simulink model "multififo"  (R2012b)
settings: Solver=ode45  StartTime=0.0  StopTime=40000  RelTol=1e-3
libraries: xbsIndex_r4 x136, xps_library x1
settings Model: Creator=tmadden  LastModifiedBy=tmadden

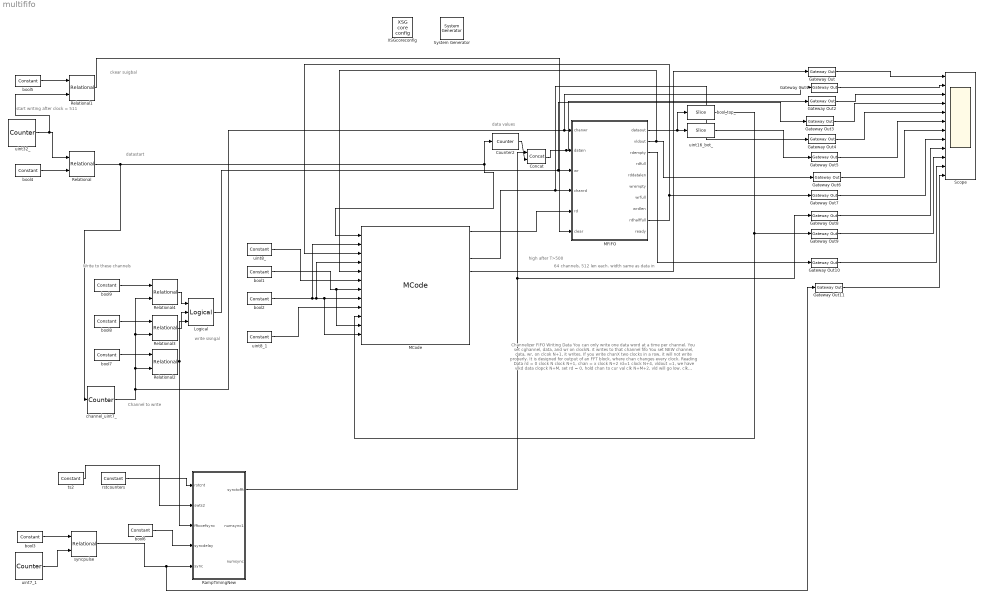
== system multififo ==
  note: Write to these channels
  note: write sisngal
  note: Channel to write
  note: data values
  note: ckear suigbal
  note: datastart
  note: start writing after clock = 511
  note: Channelizer FIFO
      | Writing Data
      | You can only write one data word at a time per channel.
      | You set cghannel, data, and wr on clockN. it writes to that channel fifo
      | You set NEW channel, data, wr, on clcok N+1, it writes.
      | If you write chanX two clocks in a row, it will not write properly.
      | It is designed for output of an FFT block, where chan changes every clock.
      |
      |
      | Reading Data
      | rd = 0 clock N
      | clock N+1, chan = x
      | clock N+2 rd=1
      | clock N+4, vldout =1, we have vlkd data
      | clopck N+M, set rd = 0, hold chan to cur val
      |
      | clk N+M+2, vld will go low.
      | clk N+M+3, chan  = new channel
      | clk N+M+4, rd=1
      | clk N+M+6, vld will be hi w/ new data
      |
      | You cannot read differnet channels per clock. you must read many data per clock,
      | at least 4 clks, so chan changes w./ rd off, and you waot for vld to go hi, 2 clkcs later.
  note: high after T>500
  note: 64 channels, 512 len each. width same as data in
  " System Generator" : xbsIndex_r4/ System Generator  Tag=genX  xilinxfamily=Kintex7  part=xc7k325t  speed=-3  package=fbg676  synthesis_tool=XST  clock_wrapper=Clock Enables  directory=./netlist  proj_type=Project Navigator  Synth_file=XST Defaults  Impl_file=ISE Defaults  testbench=off  simulink_period=1  sysclk_period=10  dcm_input_clock_period=10  incr_netlist=off  trim_vbits=Everywhere in SubSystem  dbl_ovrd=According to Block Masks  core_generation=According to Block Masks  run_coregen=off  deprecated_control=off  eval_field=0  block_type=sysgen
  Concat : xbsIndex_r4/Concat  num_inputs=2  dbl_ovrd=off  block_type=concat
  Counter2 : xbsIndex_r4/Counter  cnt_type=Free Running  cnt_to=4  operation=Up  start_count=0  cnt_by_val=1  arith_type=Unsigned  n_bits=16  bin_pt=0  load_pin=off  rst=off  en=on  explicit_period=on  period=1  dbl_ovrd=off  use_behavioral_HDL=off  implementation=Fabric  block_type=counter
  Gateway Out{,1..11} (12 alike) : xbsIndex_r4/Gateway Out  inherit_from_input=off  hdl_port=on  timing_constraint=None  locs_specified=off  LOCs={}  UseAsDAC=off  DACChannel='1'  block_type=gatewayout
  Logical : xbsIndex_r4/Logical  logical_function=OR  inputs=3  en=off  latency=0  precision=Full  arith_type=Unsigned  n_bits=16  bin_pt=0  align_bp=on  dbl_ovrd=off  block_type=logical
  MCode : xbsIndex_r4/MCode  mfname=fifoFSMPh4  explicit_period=on  period=1  inputsTable={'boundInpExpr'=>['',''],'inputs'=>['x','y']}  outputsTable={'outputs'=>['z'],'suppressOut'=>['off']}  dbl_ovrd=off  enable_stdout=off  enable_debug=off  suppress_output=on  defparams={}  hide_port_list={}  block_type=mcode
  MFIFO : Subsystem
  RampTimingNew : Subsystem
  Relational : xbsIndex_r4/Relational  mode=a>b  en=off  latency=0  dbl_ovrd=off  block_type=relational
  Relational{1..4} (4 alike) : xbsIndex_r4/Relational  mode=a=b  en=off  latency=0  dbl_ovrd=off  block_type=relational
  Scope : Scope  NumInputPorts=12
      settings: TimeRange=109.2307692307693  YMin=0~0~0~-1~0~0~0~0~-1~0~0~0  YMax=1~1~2000~1~10~2000~1~1~1~1~1~1  SaveName=ScopeData3
  XSGcoreconfig : xps_library/XSG core config  Tag=xps:xsg  hw_sys=ROACH2:sx475t  clk_src=sys_clk  ROACH_clk_src=sys_clk  ROACH2_clk_src=sys_clk  MKDIG_clk_src=sys_clk  clk_rate=100  sample_period=1  synthesis_tool=XST
  bool1 : xbsIndex_r4/Constant  const=1  gui_display_data_type=Boolean  arith_type=Boolean  n_bits=16  bin_pt=14  preci_type=Single  exp_width=8  frac_width=24  explicit_period=on  period=1  equ=P=C  opselect=C  inp2=PCIN>>17  opr=+  inp1=P  carry=CIN  dbl_ovrd=off  block_type=constant
  bool2 : xbsIndex_r4/Constant  const=0  gui_display_data_type=Boolean  arith_type=Boolean  n_bits=16  bin_pt=14  preci_type=Single  exp_width=8  frac_width=24  explicit_period=on  period=1  equ=P=C  opselect=C  inp2=PCIN>>17  opr=+  inp1=P  carry=CIN  dbl_ovrd=off  block_type=constant
  bool3 : xbsIndex_r4/Constant  const=99  gui_display_data_type=Fixed-point  arith_type=Unsigned  n_bits=16  bin_pt=0  preci_type=Single  exp_width=8  frac_width=24  explicit_period=on  period=1  equ=P=C  opselect=C  inp2=PCIN>>17  opr=+  inp1=P  carry=CIN  dbl_ovrd=off  block_type=constant
  bool4 : xbsIndex_r4/Constant  const=1024  gui_display_data_type=Fixed-point  arith_type=Unsigned  n_bits=32  bin_pt=0  preci_type=Single  exp_width=8  frac_width=24  explicit_period=on  period=1  equ=P=C  opselect=C  inp2=PCIN>>17  opr=+  inp1=P  carry=CIN  dbl_ovrd=off  block_type=constant
  bool5 : xbsIndex_r4/Constant  const=512  gui_display_data_type=Fixed-point  arith_type=Unsigned  n_bits=32  bin_pt=0  preci_type=Single  exp_width=8  frac_width=24  explicit_period=on  period=1  equ=P=C  opselect=C  inp2=PCIN>>17  opr=+  inp1=P  carry=CIN  dbl_ovrd=off  block_type=constant
  bool6 : xbsIndex_r4/Constant  const=0  gui_display_data_type=Fixed-point  arith_type=Unsigned  n_bits=16  bin_pt=0  preci_type=Single  exp_width=8  frac_width=24  explicit_period=on  period=1  equ=P=C  opselect=C  inp2=PCIN>>17  opr=+  inp1=P  carry=CIN  dbl_ovrd=off  block_type=constant
  bool7 : xbsIndex_r4/Constant  const=0  gui_display_data_type=Fixed-point  arith_type=Unsigned  n_bits=7  bin_pt=0  preci_type=Single  exp_width=8  frac_width=24  explicit_period=on  period=1  equ=P=C  opselect=C  inp2=PCIN>>17  opr=+  inp1=P  carry=CIN  dbl_ovrd=off  block_type=constant
  bool8 : xbsIndex_r4/Constant  const=7  gui_display_data_type=Fixed-point  arith_type=Unsigned  n_bits=7  bin_pt=0  preci_type=Single  exp_width=8  frac_width=24  explicit_period=on  period=1  equ=P=C  opselect=C  inp2=PCIN>>17  opr=+  inp1=P  carry=CIN  dbl_ovrd=off  block_type=constant
  bool9 : xbsIndex_r4/Constant  const=23  gui_display_data_type=Fixed-point  arith_type=Unsigned  n_bits=7  bin_pt=0  preci_type=Single  exp_width=8  frac_width=24  explicit_period=on  period=1  equ=P=C  opselect=C  inp2=PCIN>>17  opr=+  inp1=P  carry=CIN  dbl_ovrd=off  block_type=constant
  bool_top_ : xbsIndex_r4/Slice  nbits=1  boolean_output=on  mode=Upper Bit Location + Width  bit1=0  base1=MSB of Input  bit0=0  base0=LSB of Input  dbl_ovrd=off  block_type=slice
  channel_uint7_ : xbsIndex_r4/Counter  cnt_type=Free Running  cnt_to=Inf  operation=Up  start_count=0  cnt_by_val=1  arith_type=Unsigned  n_bits=7  bin_pt=0  load_pin=off  rst=off  en=on  explicit_period=on  period=1  dbl_ovrd=off  use_behavioral_HDL=off  implementation=Fabric  block_type=counter
  rstcounters : xbsIndex_r4/Constant  const=0  gui_display_data_type=Boolean  arith_type=Boolean  n_bits=16  bin_pt=14  preci_type=Single  exp_width=8  frac_width=24  explicit_period=on  period=1  equ=P=C  opselect=C  inp2=PCIN>>17  opr=+  inp1=P  carry=CIN  dbl_ovrd=off  block_type=constant
  syncpulse : xbsIndex_r4/Relational  mode=a=b  en=off  latency=0  dbl_ovrd=off  block_type=relational
  ts2 : xbsIndex_r4/Constant  const=0  gui_display_data_type=Fixed-point  arith_type=Unsigned  n_bits=32  bin_pt=0  preci_type=Single  exp_width=8  frac_width=24  explicit_period=on  period=1  equ=P=C  opselect=C  inp2=PCIN>>17  opr=+  inp1=P  carry=CIN  dbl_ovrd=off  block_type=constant
  uint16_bot_ : xbsIndex_r4/Slice  nbits=16  boolean_output=off  mode=Lower Bit Location + Width  bit1=0  base1=LSB of Input  bit0=0  base0=LSB of Input  dbl_ovrd=off  block_type=slice
  uint32_ : xbsIndex_r4/Counter  cnt_type=Free Running  cnt_to=Inf  operation=Up  start_count=0  cnt_by_val=1  arith_type=Unsigned  n_bits=32  bin_pt=0  load_pin=off  rst=off  en=off  explicit_period=on  period=1  dbl_ovrd=off  use_behavioral_HDL=off  implementation=Fabric  block_type=counter
  uint7_1 : xbsIndex_r4/Counter  cnt_type=Count Limited  cnt_to=2123  operation=Up  start_count=0  cnt_by_val=1  arith_type=Unsigned  n_bits=16  bin_pt=0  load_pin=off  rst=off  en=off  explicit_period=on  period=1  dbl_ovrd=off  use_behavioral_HDL=off  implementation=Fabric  block_type=counter
  uint8_ : xbsIndex_r4/Constant  const=63  gui_display_data_type=Fixed-point  arith_type=Unsigned  n_bits=8  bin_pt=0  preci_type=Single  exp_width=8  frac_width=24  explicit_period=on  period=1  equ=P=C  opselect=C  inp2=PCIN>>17  opr=+  inp1=P  carry=CIN  dbl_ovrd=off  block_type=constant
  uint8_1 : xbsIndex_r4/Constant  const=129  gui_display_data_type=Fixed-point  arith_type=Unsigned  n_bits=8  bin_pt=0  preci_type=Single  exp_width=8  frac_width=24  explicit_period=on  period=1  equ=P=C  opselect=C  inp2=PCIN>>17  opr=+  inp1=P  carry=CIN  dbl_ovrd=off  block_type=constant
  wires:
  Counter2/1 -> Concat/2
  uint16_bot_/1 -> Gateway Out5/1
  MFIFO/2(vldout) -> MCode/5, Gateway Out6/1
  Gateway Out1/1 -> Scope/2
  Gateway Out2/1 -> Scope/3
  Gateway Out3/1 -> Scope/4
  Gateway Out4/1 -> Scope/5
  Gateway Out5/1 -> Scope/6
  Gateway Out6/1 -> Scope/7
  Gateway Out7/1 -> Scope/8
  Gateway Out8/1 -> Scope/9
  Gateway Out9/1 -> Scope/10
  Gateway Out10/1 -> Scope/11
  Gateway Out11/1 -> Scope/12
  MCode/3 -> Gateway Out4/1, MFIFO/4(chanrd)
  MCode/1 -> MFIFO/5(rd)
  bool2/1 -> MCode/8, MCode/12, MCode/4, MCode/2
  bool1/1 -> MCode/11, MCode/7
  uint8_/1 -> MCode/6
  uint8_1/1 -> MCode/9
  MFIFO/9(rdhalffull) -> Gateway Out7/1, MCode/3
  bool4/1 -> Relational/2
  uint32_/1 -> Relational1/2, Relational/1
  Relational/1 -> channel_uint7_/1, MCode/1, Counter2/1
  bool5/1 -> Relational1/1
  Relational1/1 -> MFIFO/6(clear)
  Gateway Out/1 -> Scope/1
  bool3/1 -> syncpulse/1
  uint7_1/1 -> syncpulse/2
  RampTimingNew/1(synctofft) -> Gateway Out8/1, Concat/1
  MFIFO/1(dataout) -> bool_top_/1, uint16_bot_/1
  bool_top_/1 -> Gateway Out9/1, MCode/10
  MCode/4 -> Gateway Out/1
  MFIFO/3(rdempty) -> Gateway Out10/1
  syncpulse/1 -> Gateway Out11/1, RampTimingNew/5(sync)
  bool6/1 -> RampTimingNew/4(syncdelay)
  rstcounters/1 -> RampTimingNew/1(rstcnt)
  ts2/1 -> RampTimingNew/2(swts2)
  bool9/1 -> Relational4/1
  bool8/1 -> Relational3/1
  bool7/1 -> Relational2/1
  channel_uint7_/1 -> Gateway Out1/1, MFIFO/1(chanwr), Relational2/2, Relational3/2, Relational4/2
  Relational4/1 -> Logical/1
  Relational3/1 -> Logical/2
  Relational2/1 -> RampTimingNew/3(fftcoefsync), Logical/3
  Logical/1 -> MFIFO/3(wr), Gateway Out3/1
  Concat/1 -> Gateway Out2/1, MFIFO/2(datain)

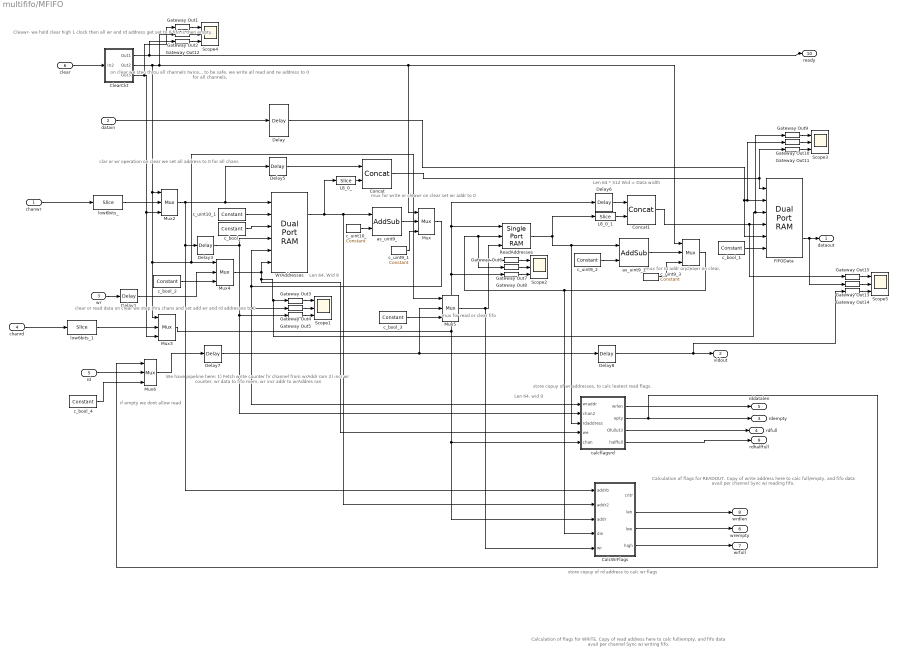
== system multififo/MFIFO ==
  note: store copuy of rd address to calc wr flags
  note: store copuy of wr addresses, to calc leatest read flags.
  note: on clear we steo throu all channels
      | twice... to be safe.
      | we write all read and rw address to 0 for all channels.
  note: clar or wr operation
      | on clear we set all address to 0 for all chans
  note: clear or read data
      | on clear we step thru chans and
      | set add wr and rd addresses to 0
  note: mux for rd addr or cleawr
      | on clear,
  note: mux for write or cleawr
      | on clear set wr addr to 0
  note: mux for read or clear fifo
  note: if empty we dont allow read
  note: Cleawr- we hold clear high 1 clock
      | then all wr and rd address get set to 0
      | fifo is then empty.
  note: Calculation of flags for READOUT.
      | Copy of write address here to calc full/empty, and fifo
      | data avail per channel
      | Sync w/ reading fifo.
  note: Len 64 * 512
      | Wid = Data width
  note: Len 64, wid 9
  note: Len 64, Wid 9
  note: We have pipeline here:
      | 1) Fetch write counter fir channel from wrAddr ram
      | 2) incr wr counter, wr data to fifo mem, wr incr addr to wrAddres ran
  note: Calculation of flags for WRITE.
      | Copy of read address here to calc full/empty, and fifo
      | data avail per channel
      | Sync w/ writing fifo.
  chanwr : Inport
  datain : Inport  Port=2
  wr : Inport  Port=3
  chanrd : Inport  Port=4
  rd : Inport  Port=5
  clear : Inport  Port=6
  CalcWrFlags : Subsystem
  ClearCkt : Subsystem
  Concat : xbsIndex_r4/Concat  num_inputs=2  dbl_ovrd=off  block_type=concat
  Concat1 : xbsIndex_r4/Concat  num_inputs=2  dbl_ovrd=off  block_type=concat
  Delay{,1,3,5..8} (7 alike) : xbsIndex_r4/Delay  rst=off  infoeditControl=Selection of Reset will increase slice count due to use of real FFs and instead of SRLs  en=off  latency=1  dbl_ovrd=off  reg_retiming=off  block_type=delay
  FIFOData : xbsIndex_r4/Dual Port RAM  depth=32768  initVector=zeros(1,32768)  distributed_mem=Block RAM  init_a=0  init_b=0  rst_a=off  rst_b=off  en_a=off  en_b=off  latency=1  write_mode_A=Read Before Write  write_mode_B=Read Before Write  dbl_ovrd=off  optimize=Speed  block_type=dpram
  Gateway Out{1..15} (15 alike) : xbsIndex_r4/Gateway Out  inherit_from_input=off  hdl_port=on  timing_constraint=None  locs_specified=off  LOCs={}  UseAsDAC=off  DACChannel='1'  block_type=gatewayout
  L8_0_ : xbsIndex_r4/Slice  nbits=9  boolean_output=off  mode=Lower Bit Location + Width  bit1=0  base1=MSB of Input  bit0=0  base0=LSB of Input  dbl_ovrd=off  block_type=slice
  L8_0_1 : xbsIndex_r4/Slice  nbits=9  boolean_output=off  mode=Lower Bit Location + Width  bit1=0  base1=MSB of Input  bit0=0  base0=LSB of Input  dbl_ovrd=off  block_type=slice
  Mux{,1..6} (7 alike) : xbsIndex_r4/Mux  inputs=2  en=off  latency=0  precision=Full  arith_type=Unsigned  n_bits=16  bin_pt=14  quantization=Truncate  overflow=Wrap  dbl_ovrd=off  block_type=mux
  ReadAddresses : xbsIndex_r4/Single Port RAM  depth=64  initVector=zeros(1,64)  distributed_mem=Block RAM  write_mode=Read After Write  rst=off  init_reg=0  en=off  latency=1  dbl_ovrd=off  optimize=Speed  block_type=spram
  Scope{1..5} (5 alike) : Scope  NumInputPorts=3
      Scope1 settings: YMin=-5~-5~-5  YMax=5~5~5
      Scope2 settings: YMin=-5~-5~-5  YMax=5~5~5  SaveName=ScopeData2
      Scope3 settings: YMin=-5~-5~-5  YMax=5~5~5  SaveName=ScopeData4
      Scope4 settings: YMin=-5~-5~-5  YMax=5~5~5
      Scope5 settings: YMin=-5~-5~-5  YMax=5~5~5  SaveName=ScopeData7
  WrAddresses : xbsIndex_r4/Dual Port RAM  depth=64  initVector=zeros(1,64)  distributed_mem=Block RAM  init_a=0  init_b=0  rst_a=off  rst_b=off  en_a=off  en_b=off  latency=1  write_mode_A=Read Before Write  write_mode_B=Read Before Write  dbl_ovrd=off  optimize=Speed  block_type=dpram
  as_uint9_ : xbsIndex_r4/AddSub  mode=Addition  use_carryin=off  use_carryout=off  en=off  latency=0  precision=User Defined  arith_type=Unsigned  n_bits=10  bin_pt=0  quantization=Truncate  overflow=Wrap  dbl_ovrd=off  use_behavioral_HDL=off  hw_selection=Fabric  pipelined=off  block_type=addsub
  as_uint9_1 : xbsIndex_r4/AddSub  mode=Addition  use_carryin=off  use_carryout=off  en=off  latency=0  precision=User Defined  arith_type=Unsigned  n_bits=10  bin_pt=0  quantization=Truncate  overflow=Wrap  dbl_ovrd=off  use_behavioral_HDL=off  hw_selection=Fabric  pipelined=off  block_type=addsub
  c_bool_ : xbsIndex_r4/Constant  const=0  gui_display_data_type=Boolean  arith_type=Boolean  n_bits=9  bin_pt=0  preci_type=Single  exp_width=8  frac_width=24  explicit_period=on  period=1  equ=P=C  opselect=C  inp2=PCIN>>17  opr=+  inp1=P  carry=CIN  dbl_ovrd=off  block_type=constant
  c_bool_1 : xbsIndex_r4/Constant  const=0  gui_display_data_type=Boolean  arith_type=Boolean  n_bits=9  bin_pt=0  preci_type=Single  exp_width=8  frac_width=24  explicit_period=on  period=1  equ=P=C  opselect=C  inp2=PCIN>>17  opr=+  inp1=P  carry=CIN  dbl_ovrd=off  block_type=constant
  c_bool_2 : xbsIndex_r4/Constant  const=1  gui_display_data_type=Boolean  arith_type=Boolean  n_bits=9  bin_pt=0  preci_type=Single  exp_width=8  frac_width=24  explicit_period=on  period=1  equ=P=C  opselect=C  inp2=PCIN>>17  opr=+  inp1=P  carry=CIN  dbl_ovrd=off  block_type=constant
  c_bool_3 : xbsIndex_r4/Constant  const=1  gui_display_data_type=Boolean  arith_type=Boolean  n_bits=9  bin_pt=0  preci_type=Single  exp_width=8  frac_width=24  explicit_period=on  period=1  equ=P=C  opselect=C  inp2=PCIN>>17  opr=+  inp1=P  carry=CIN  dbl_ovrd=off  block_type=constant
  c_bool_4 : xbsIndex_r4/Constant  const=0  gui_display_data_type=Boolean  arith_type=Boolean  n_bits=9  bin_pt=0  preci_type=Single  exp_width=8  frac_width=24  explicit_period=on  period=1  equ=P=C  opselect=C  inp2=PCIN>>17  opr=+  inp1=P  carry=CIN  dbl_ovrd=off  block_type=constant
  c_uint10_ : xbsIndex_r4/Constant  const=1  gui_display_data_type=Fixed-point  arith_type=Unsigned  n_bits=10  bin_pt=0  preci_type=Single  exp_width=8  frac_width=24  explicit_period=on  period=1  equ=P=C  opselect=C  inp2=PCIN>>17  opr=+  inp1=P  carry=CIN  dbl_ovrd=off  block_type=constant
  c_uint10_1 : xbsIndex_r4/Constant  const=0  gui_display_data_type=Fixed-point  arith_type=Unsigned  n_bits=10  bin_pt=0  preci_type=Single  exp_width=8  frac_width=24  explicit_period=on  period=1  equ=P=C  opselect=C  inp2=PCIN>>17  opr=+  inp1=P  carry=CIN  dbl_ovrd=off  block_type=constant
  c_uint9_1 : xbsIndex_r4/Constant  const=0  gui_display_data_type=Fixed-point  arith_type=Unsigned  n_bits=10  bin_pt=0  preci_type=Single  exp_width=8  frac_width=24  explicit_period=on  period=1  equ=P=C  opselect=C  inp2=PCIN>>17  opr=+  inp1=P  carry=CIN  dbl_ovrd=off  block_type=constant
  c_uint9_2 : xbsIndex_r4/Constant  const=1  gui_display_data_type=Fixed-point  arith_type=Unsigned  n_bits=10  bin_pt=0  preci_type=Single  exp_width=8  frac_width=24  explicit_period=on  period=1  equ=P=C  opselect=C  inp2=PCIN>>17  opr=+  inp1=P  carry=CIN  dbl_ovrd=off  block_type=constant
  c_uint9_3 : xbsIndex_r4/Constant  const=0  gui_display_data_type=Fixed-point  arith_type=Unsigned  n_bits=10  bin_pt=0  preci_type=Single  exp_width=8  frac_width=24  explicit_period=on  period=1  equ=P=C  opselect=C  inp2=PCIN>>17  opr=+  inp1=P  carry=CIN  dbl_ovrd=off  block_type=constant
  calcflagsrd : Subsystem
  low6bits_ : xbsIndex_r4/Slice  nbits=6  boolean_output=off  mode=Lower Bit Location + Width  bit1=0  base1=MSB of Input  bit0=0  base0=LSB of Input  dbl_ovrd=off  block_type=slice
  low6bits_1 : xbsIndex_r4/Slice  nbits=6  boolean_output=off  mode=Lower Bit Location + Width  bit1=0  base1=MSB of Input  bit0=0  base0=LSB of Input  dbl_ovrd=off  block_type=slice
  dataout : Outport
  vldout : Outport  Port=2
  rdempty : Outport  Port=3
  rdfull : Outport  Port=4
  rddatalen : Outport  Port=5
  wrempty : Outport  Port=6
  wrfull : Outport  Port=7
  wrdlen : Outport  Port=8
  rdhalffull : Outport  Port=9
  ready : Outport  Port=10
  wires:
  Concat/1 -> FIFOData/1, Gateway Out11/1
  Delay/1 -> FIFOData/5, Gateway Out10/1, FIFOData/2
  Delay5/1 -> Concat/1
  Delay8/1 -> Gateway Out14/1, vldout/1
  Mux6/1 -> Delay7/1
  chanwr/1 -> low6bits_/1
  Mux3/1 -> Delay6/1, ReadAddresses/1, Gateway Out8/1, CalcWrFlags/3(addr), calcflagsrd/5(chan)
  Delay6/1 -> Concat1/1
  Delay1/1 -> Mux4/2
  Delay3/1 -> Gateway Out5/1, calcflagsrd/2(chan2), WrAddresses/4
  c_bool_1/1 -> FIFOData/6
  Mux1/1 -> CalcWrFlags/4(din), Gateway Out7/1, ReadAddresses/2
  c_uint9_2/1 -> as_uint9_1/2
  Mux/1 -> Gateway Out4/1, calcflagsrd/1(wraddr), WrAddresses/5
  Concat1/1 -> Gateway Out15/1, FIFOData/4
  wr/1 -> Delay1/1
  datain/1 -> Delay/1
  Delay7/1 -> Mux5/2, Delay8/1
  c_uint10_/1 -> as_uint9_/2
  WrAddresses/1 -> L8_0_/1, CalcWrFlags/2(addr2), as_uint9_/1
  FIFOData/2 -> Gateway Out13/1, dataout/1
  L8_0_/1 -> Concat/2
  L8_0_1/1 -> Concat1/2
  c_uint10_1/1 -> WrAddresses/2
  c_bool_/1 -> WrAddresses/3
  ReadAddresses/1 -> as_uint9_1/1, calcflagsrd/3(rdaddress), L8_0_1/1
  Mux2/1 -> Delay3/1, CalcWrFlags/1(addrb), WrAddresses/1, Delay5/1
  CalcWrFlags/2(len) -> wrdlen/1
  CalcWrFlags/3(low) -> wrempty/1
  CalcWrFlags/4(high) -> wrfull/1
  calcflagsrd/1(wrlen) -> rddatalen/1
  calcflagsrd/2(epty) -> Mux6/1, rdempty/1
  calcflagsrd/3(Ofullut3) -> rdfull/1
  calcflagsrd/4(halffull) -> rdhalffull/1
  as_uint9_/1 -> Mux/2
  c_uint9_1/1 -> Mux/3
  as_uint9_1/1 -> Mux1/2
  c_uint9_3/1 -> Mux1/3
  low6bits_/1 -> Mux2/2
  ClearCkt/3(Out3) -> Gateway Out12/1, Mux3/3, Mux2/3
  ClearCkt/2(Out2) -> Gateway Out2/1, Mux1/1, Mux/1, Mux4/1, Mux5/1, Mux3/1, Mux2/1
  clear/1 -> ClearCkt/1(In2)
  ClearCkt/1(Out1) -> Gateway Out1/1, ready/1
  Gateway Out5/1 -> Scope1/3
  Gateway Out4/1 -> Scope1/2
  Gateway Out3/1 -> Scope1/1
  Gateway Out8/1 -> Scope2/3
  Gateway Out7/1 -> Scope2/2
  Gateway Out6/1 -> Scope2/1
  Gateway Out11/1 -> Scope3/3
  Gateway Out10/1 -> Scope3/2
  Gateway Out9/1 -> Scope3/1
  Gateway Out12/1 -> Scope4/3
  Gateway Out2/1 -> Scope4/2
  Gateway Out1/1 -> Scope4/1
  Mux4/1 -> calcflagsrd/4(we), Gateway Out9/1, FIFOData/3, Gateway Out3/1, WrAddresses/6
  c_bool_2/1 -> Mux4/3
  c_bool_3/1 -> Mux5/3
  Mux5/1 -> CalcWrFlags/5(wr), Gateway Out6/1, ReadAddresses/3
  Gateway Out14/1 -> Scope5/3
  Gateway Out13/1 -> Scope5/2
  Gateway Out15/1 -> Scope5/1
  rd/1 -> Mux6/2
  c_bool_4/1 -> Mux6/3
  low6bits_1/1 -> Mux3/2
  chanrd/1 -> low6bits_1/1

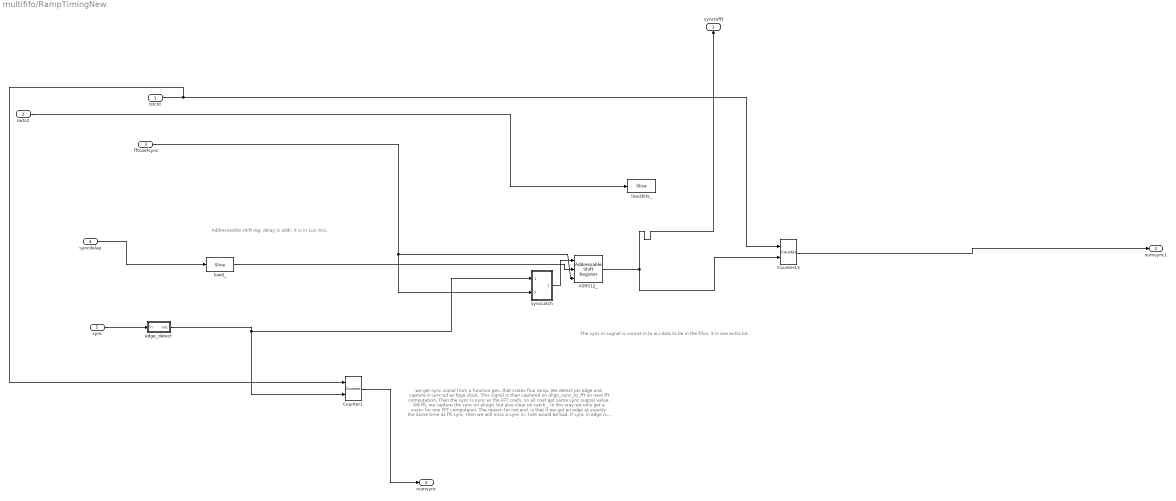
== system multififo/RampTimingNew ==
  note: Addressavble shift reg.
      | delay is addr. it is in 1us incs.
  note: The sync in sugnal is
      | concat in to w./ data to
      | be in the fifos.
      | it is one extra bit.
  note: we get sync signal from a function gen, that crates flux ramp.
      | We detect pls edge and capture it  sync'ed w/ fpga clock.
      | This signal is than captured on align_sunc_to_fft on next fft
      | computation. Then the sync is sync w/ the FFT coefs, so all coef get same
      | sync sugnal value.
      | ON fft, we capture the sync on aliogn, but also clear on catch_. In this way
      | we only get a suync for one FFT computaion.
      | The reason for not and, is that if we get an edge at exactly the same time
      | as fft sync, then we will miss a sync in. Taht would be bad.
      | If sync in edge is high, we won't reset the catch-sync, but catch it.
      | FFT coef sync runs at 1MHz. sunc in should be at less then 100kHz
      | so there should be no way we would MISS resetting the catch_
      | As long as fft_coef sync is faster than sync in,this should work.
  rstcnt : Inport
  swts2 : Inport  Port=2
  fftcoefsync : Inport  Port=3
  syncdelay : Inport  Port=4
  sync : Inport  Port=5
  ASR512_ : xbsIndex_r4/Addressable Shift Register  infer_latency=off  depth=256  initVector=[0]  en=on  dbl_ovrd=off  use_behavioral_HDL=off  Optimization=Resource  block_type=addrsr
      settings: infoedit="Delay of configurable length.  Any element in the delay line can be addressed and driven onto the output port.<br><br>Hardware notes: This block is implemented using SRL16s. If Virtex-4 or Spartan-3 device is used, multiple SRLC16s are cascaded together."
  Counter1 : xbsIndex_r4/Counter  cnt_type=Free Running  cnt_to=Inf  operation=Up  start_count=0  cnt_by_val=1  arith_type=Unsigned  n_bits=32  bin_pt=0  load_pin=off  rst=on  en=on  explicit_period=on  period=1  dbl_ovrd=off  use_behavioral_HDL=off  implementation=Fabric  block_type=counter
  Counter13 : xbsIndex_r4/Counter  cnt_type=Free Running  cnt_to=Inf  operation=Up  start_count=0  cnt_by_val=1  arith_type=Unsigned  n_bits=32  bin_pt=0  load_pin=off  rst=on  en=on  explicit_period=on  period=1  dbl_ovrd=off  use_behavioral_HDL=off  implementation=Fabric  block_type=counter
  edge_detect : Subsystem  AncestorBlock=casper_library_misc/edge_detect  mask(edge_detect){edge=Rising, polarity=Active High, x_in=[0 0.08 0.08 0.16 0.16 0.24 0.24 0.32 0.32 0.4], y_in=[-1 -1  1  1  1  1  1  1  1  1], x_out=[0.6 0.68 0.68 0.76 0.76 0.84 0.84 0.92 0.92 1], y_out=[-1 -1  1  1 -1 -1 -1 -1 -1 -1]}
      mask prompts: edge "Edge Type"; polarity "Output Polarity"; x_in "Input X Positions"; y_in "Input Y Positions"; x_out "Output X Positions"; y_out "Output Y Positions"
      mask help: Output is active for one-cycle after each edge of the specified type (i.e. rising, falling or both).
      mask init:
      | edge_detect_init(gcb,...
      |     'edge',edge,...
      |     'polarity',polarity,...
      |     'x_in',x_in,...
      |     'x_out',x_out,...
      |     'y_in',y_in,...
      |     'y_out',y_out);
      | 
      | x_in_num=str2num(getfield(getfield(get_param(gcb,'UserData'),'parameters'),'x_in'));
      | x_out_num=str2num(getfield(getfield(get_param(gcb,'UserData'),'parameters'),'x_out'));
      | y_in_num=str2num(getfield(getfield(get_param(gcb,'UserData'),'parameters'),'y_in'));
      | y_out_num=str2num(getfield(getfield(get_param(gcb,'UserData'),'parameters'),'y_out'));
      settings: AttributesFormatString=|
      | rising edges
      | active high
      mask Help: Output is active for one-cycle after each edge of the specified type (i.e. rising, falling, or both).  Latency is zero.
      mask TypeOptions edge: Rising | Falling | Both
      mask TypeOptions polarity: Active High | Active Low
      mask Display:
      | plot(x_in_num,0.5+y_in_num*0.2);
      | plot(x_out_num,0.5+y_out_num*0.2);
  low2bits_ : xbsIndex_r4/Slice  nbits=2  boolean_output=off  mode=Lower Bit Location + Width  bit1=0  base1=MSB of Input  bit0=0  base0=LSB of Input  dbl_ovrd=off  block_type=slice
  low8_ : xbsIndex_r4/Slice  nbits=8  boolean_output=off  mode=Lower Bit Location + Width  bit1=0  base1=MSB of Input  bit0=0  base0=LSB of Input  dbl_ovrd=off  block_type=slice
  synccatch : Subsystem
  synctofft : Outport
  numsync1 : Outport  Port=2
  numsync : Outport  Port=3
  wires:
  fftcoefsync/1 -> ASR512_/3, synccatch/2(fftcoefsync)
  syncdelay/1 -> low8_/1
  edge_detect/1(out) -> synccatch/1(syncpulse), Counter1/2
  Counter1/1 -> numsync/1
  rstcnt/1 -> Counter1/1, Counter13/1
  Counter13/1 -> numsync1/1
  sync/1 -> edge_detect/1(in)
  swts2/1 -> low2bits_/1
  ASR512_/1 -> synctofft/1, Counter13/2
  synccatch/1(Out1) -> ASR512_/1
  low8_/1 -> ASR512_/2

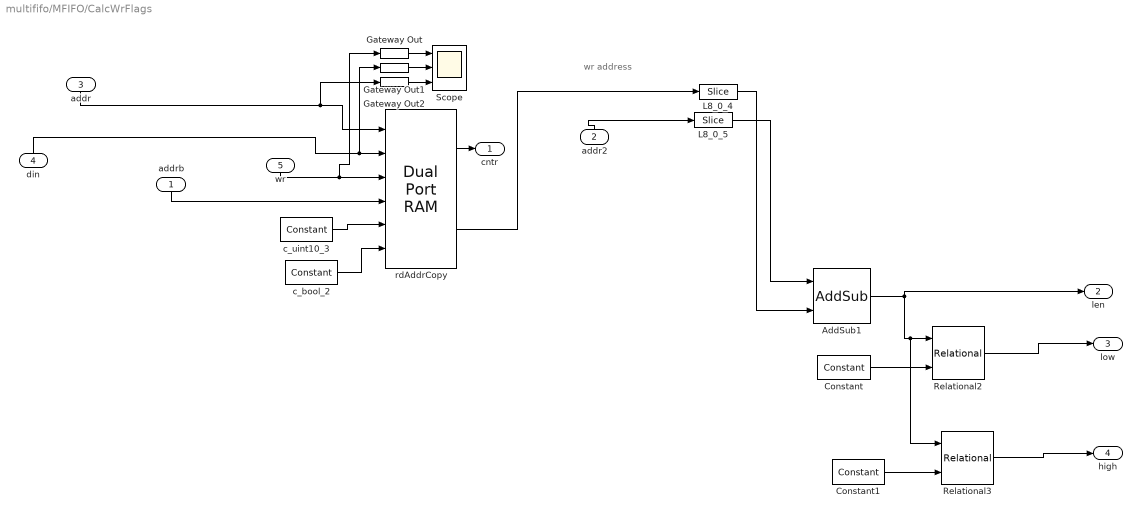
== system multififo/MFIFO/CalcWrFlags ==
  note: wr address
  addrb : Inport
  addr2 : Inport  Port=2
  addr : Inport  Port=3
  din : Inport  Port=4
  wr : Inport  Port=5
  AddSub1 : xbsIndex_r4/AddSub  mode=Subtraction  use_carryin=off  use_carryout=off  en=off  latency=0  precision=User Defined  arith_type=Unsigned  n_bits=9  bin_pt=0  quantization=Truncate  overflow=Wrap  dbl_ovrd=off  use_behavioral_HDL=off  hw_selection=Fabric  pipelined=off  block_type=addsub
  Constant : xbsIndex_r4/Constant  const=8  gui_display_data_type=Fixed-point  arith_type=Unsigned  n_bits=9  bin_pt=0  preci_type=Single  exp_width=8  frac_width=24  explicit_period=on  period=1  equ=P=C  opselect=C  inp2=PCIN>>17  opr=+  inp1=P  carry=CIN  dbl_ovrd=off  block_type=constant
  Constant1 : xbsIndex_r4/Constant  const=503  gui_display_data_type=Fixed-point  arith_type=Unsigned  n_bits=9  bin_pt=0  preci_type=Single  exp_width=8  frac_width=24  explicit_period=on  period=1  equ=P=C  opselect=C  inp2=PCIN>>17  opr=+  inp1=P  carry=CIN  dbl_ovrd=off  block_type=constant
  Gateway Out : xbsIndex_r4/Gateway Out  inherit_from_input=off  hdl_port=on  timing_constraint=None  locs_specified=off  LOCs={}  UseAsDAC=off  DACChannel='1'  block_type=gatewayout
  Gateway Out1 : xbsIndex_r4/Gateway Out  inherit_from_input=off  hdl_port=on  timing_constraint=None  locs_specified=off  LOCs={}  UseAsDAC=off  DACChannel='1'  block_type=gatewayout
  Gateway Out2 : xbsIndex_r4/Gateway Out  inherit_from_input=off  hdl_port=on  timing_constraint=None  locs_specified=off  LOCs={}  UseAsDAC=off  DACChannel='1'  block_type=gatewayout
  L8_0_4 : xbsIndex_r4/Slice  nbits=9  boolean_output=off  mode=Lower Bit Location + Width  bit1=0  base1=MSB of Input  bit0=0  base0=LSB of Input  dbl_ovrd=off  block_type=slice
  L8_0_5 : xbsIndex_r4/Slice  nbits=9  boolean_output=off  mode=Lower Bit Location + Width  bit1=0  base1=MSB of Input  bit0=0  base0=LSB of Input  dbl_ovrd=off  block_type=slice
  Relational2 : xbsIndex_r4/Relational  mode=a<b  en=off  latency=0  dbl_ovrd=off  block_type=relational
  Relational3 : xbsIndex_r4/Relational  mode=a>b  en=off  latency=0  dbl_ovrd=off  block_type=relational
  Scope : Scope  NumInputPorts=3
      settings: YMin=-5~-5~-5  YMax=5~5~5  SaveName=ScopeData6
  c_bool_2 : xbsIndex_r4/Constant  const=0  gui_display_data_type=Boolean  arith_type=Boolean  n_bits=9  bin_pt=0  preci_type=Single  exp_width=8  frac_width=24  explicit_period=on  period=1  equ=P=C  opselect=C  inp2=PCIN>>17  opr=+  inp1=P  carry=CIN  dbl_ovrd=off  block_type=constant
  c_uint10_3 : xbsIndex_r4/Constant  const=0  gui_display_data_type=Fixed-point  arith_type=Unsigned  n_bits=10  bin_pt=0  preci_type=Single  exp_width=8  frac_width=24  explicit_period=on  period=1  equ=P=C  opselect=C  inp2=PCIN>>17  opr=+  inp1=P  carry=CIN  dbl_ovrd=off  block_type=constant
  rdAddrCopy : xbsIndex_r4/Dual Port RAM  depth=64  initVector=zeros(1,64)  distributed_mem=Block RAM  init_a=0  init_b=0  rst_a=off  rst_b=off  en_a=off  en_b=off  latency=1  write_mode_A=Read Before Write  write_mode_B=Read Before Write  dbl_ovrd=off  optimize=Speed  block_type=dpram
  cntr : Outport
  len : Outport  Port=2
  low : Outport  Port=3
  high : Outport  Port=4
  wires:
  L8_0_4/1 -> AddSub1/2
  Constant/1 -> Relational2/2
  rdAddrCopy/2 -> L8_0_4/1
  addr/1 -> Gateway Out2/1, rdAddrCopy/1
  addrb/1 -> rdAddrCopy/4
  addr2/1 -> L8_0_5/1
  AddSub1/1 -> len/1, Relational3/1, Relational2/1
  c_uint10_3/1 -> rdAddrCopy/5
  Relational2/1 -> low/1
  din/1 -> Gateway Out1/1, rdAddrCopy/2
  wr/1 -> Gateway Out/1, rdAddrCopy/3
  Relational3/1 -> high/1
  L8_0_5/1 -> AddSub1/1
  c_bool_2/1 -> rdAddrCopy/6
  Constant1/1 -> Relational3/2
  rdAddrCopy/1 -> cntr/1
  Gateway Out2/1 -> Scope/3
  Gateway Out1/1 -> Scope/2
  Gateway Out/1 -> Scope/1

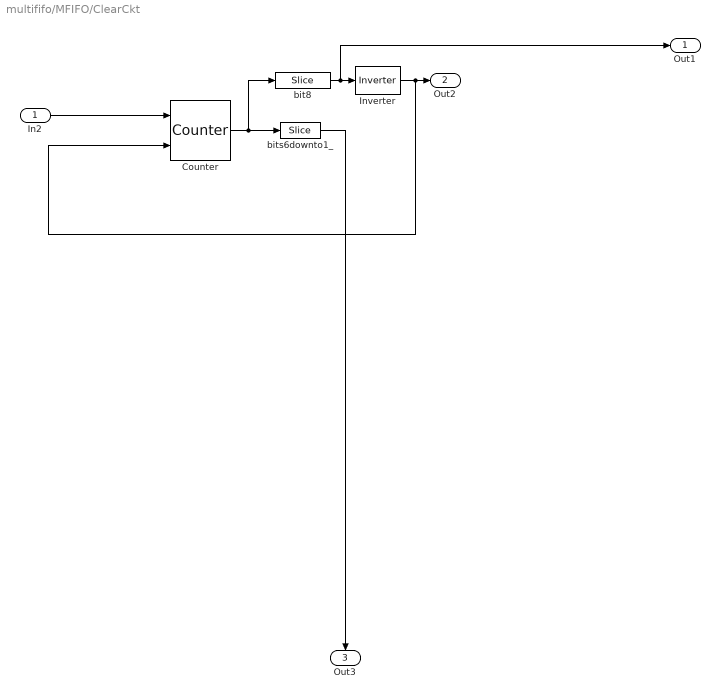
== system multififo/MFIFO/ClearCkt ==
  In2 : Inport
  Counter : xbsIndex_r4/Counter  cnt_type=Free Running  cnt_to=Inf  operation=Up  start_count=0  cnt_by_val=1  arith_type=Unsigned  n_bits=9  bin_pt=0  load_pin=off  rst=on  en=on  explicit_period=on  period=1  dbl_ovrd=off  use_behavioral_HDL=off  implementation=Fabric  block_type=counter
  Inverter : xbsIndex_r4/Inverter  en=off  latency=0  dbl_ovrd=off  block_type=inv
  bit8 : xbsIndex_r4/Slice  nbits=1  boolean_output=on  mode=Upper Bit Location + Width  bit1=0  base1=MSB of Input  bit0=0  base0=LSB of Input  dbl_ovrd=off  block_type=slice
  bits6downto1_ : xbsIndex_r4/Slice  nbits=6  boolean_output=off  mode=Lower Bit Location + Width  bit1=0  base1=MSB of Input  bit0=1  base0=LSB of Input  dbl_ovrd=off  block_type=slice
  Out1 : Outport
  Out2 : Outport  Port=2
  Out3 : Outport  Port=3
  wires:
  Counter/1 -> bit8/1, bits6downto1_/1
  In2/1 -> Counter/1
  bit8/1 -> Out1/1, Inverter/1
  bits6downto1_/1 -> Out3/1
  Inverter/1 -> Counter/2, Out2/1

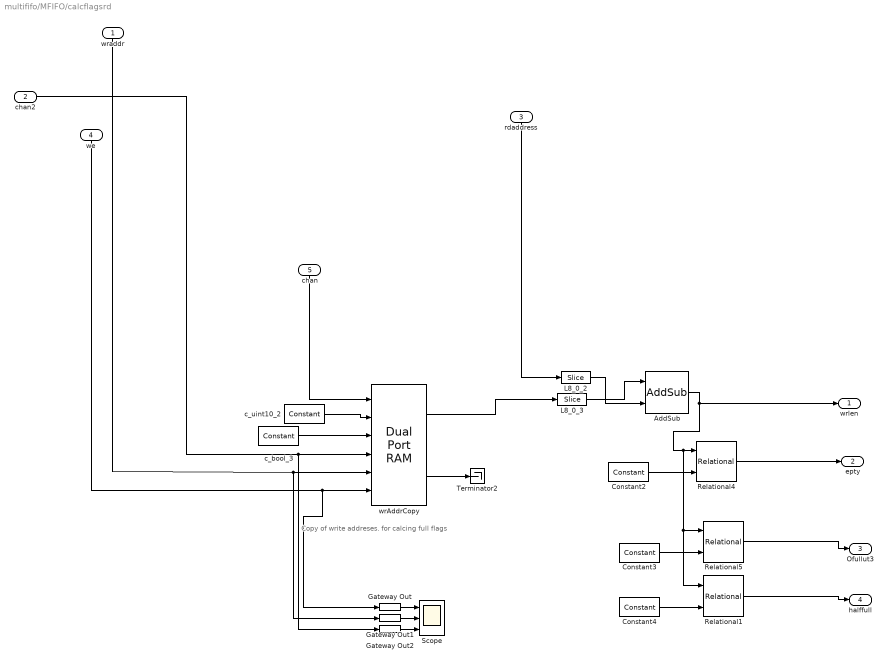
== system multififo/MFIFO/calcflagsrd ==
  note: Copy of write addreses. for calcing full flags
  wraddr : Inport
  chan2 : Inport  Port=2
  rdaddress : Inport  Port=3
  we : Inport  Port=4
  chan : Inport  Port=5
  AddSub : xbsIndex_r4/AddSub  mode=Subtraction  use_carryin=off  use_carryout=off  en=off  latency=0  precision=User Defined  arith_type=Unsigned  n_bits=9  bin_pt=0  quantization=Truncate  overflow=Wrap  dbl_ovrd=off  use_behavioral_HDL=off  hw_selection=Fabric  pipelined=off  block_type=addsub
  Constant2 : xbsIndex_r4/Constant  const=8  gui_display_data_type=Fixed-point  arith_type=Unsigned  n_bits=9  bin_pt=0  preci_type=Single  exp_width=8  frac_width=24  explicit_period=on  period=1  equ=P=C  opselect=C  inp2=PCIN>>17  opr=+  inp1=P  carry=CIN  dbl_ovrd=off  block_type=constant
  Constant3 : xbsIndex_r4/Constant  const=503  gui_display_data_type=Fixed-point  arith_type=Unsigned  n_bits=9  bin_pt=0  preci_type=Single  exp_width=8  frac_width=24  explicit_period=on  period=1  equ=P=C  opselect=C  inp2=PCIN>>17  opr=+  inp1=P  carry=CIN  dbl_ovrd=off  block_type=constant
  Constant4 : xbsIndex_r4/Constant  const=384  gui_display_data_type=Fixed-point  arith_type=Unsigned  n_bits=9  bin_pt=0  preci_type=Single  exp_width=8  frac_width=24  explicit_period=on  period=1  equ=P=C  opselect=C  inp2=PCIN>>17  opr=+  inp1=P  carry=CIN  dbl_ovrd=off  block_type=constant
  Gateway Out : xbsIndex_r4/Gateway Out  inherit_from_input=off  hdl_port=on  timing_constraint=None  locs_specified=off  LOCs={}  UseAsDAC=off  DACChannel='1'  block_type=gatewayout
  Gateway Out1 : xbsIndex_r4/Gateway Out  inherit_from_input=off  hdl_port=on  timing_constraint=None  locs_specified=off  LOCs={}  UseAsDAC=off  DACChannel='1'  block_type=gatewayout
  Gateway Out2 : xbsIndex_r4/Gateway Out  inherit_from_input=off  hdl_port=on  timing_constraint=None  locs_specified=off  LOCs={}  UseAsDAC=off  DACChannel='1'  block_type=gatewayout
  L8_0_2 : xbsIndex_r4/Slice  nbits=9  boolean_output=off  mode=Lower Bit Location + Width  bit1=0  base1=MSB of Input  bit0=0  base0=LSB of Input  dbl_ovrd=off  block_type=slice
  L8_0_3 : xbsIndex_r4/Slice  nbits=9  boolean_output=off  mode=Lower Bit Location + Width  bit1=0  base1=MSB of Input  bit0=0  base0=LSB of Input  dbl_ovrd=off  block_type=slice
  Relational1 : xbsIndex_r4/Relational  mode=a>b  en=off  latency=0  dbl_ovrd=off  block_type=relational
  Relational4 : xbsIndex_r4/Relational  mode=a<b  en=off  latency=0  dbl_ovrd=off  block_type=relational
  Relational5 : xbsIndex_r4/Relational  mode=a>b  en=off  latency=0  dbl_ovrd=off  block_type=relational
  Scope : Scope  NumInputPorts=3
      settings: YMin=-5~-5~-5  YMax=5~5~5  SaveName=ScopeData5
  Terminator2 : Terminator
  c_bool_3 : xbsIndex_r4/Constant  const=0  gui_display_data_type=Boolean  arith_type=Boolean  n_bits=9  bin_pt=0  preci_type=Single  exp_width=8  frac_width=24  explicit_period=on  period=1  equ=P=C  opselect=C  inp2=PCIN>>17  opr=+  inp1=P  carry=CIN  dbl_ovrd=off  block_type=constant
  c_uint10_2 : xbsIndex_r4/Constant  const=0  gui_display_data_type=Fixed-point  arith_type=Unsigned  n_bits=10  bin_pt=0  preci_type=Single  exp_width=8  frac_width=24  explicit_period=on  period=1  equ=P=C  opselect=C  inp2=PCIN>>17  opr=+  inp1=P  carry=CIN  dbl_ovrd=off  block_type=constant
  wrAddrCopy : xbsIndex_r4/Dual Port RAM  depth=64  initVector=zeros(1,64)  distributed_mem=Block RAM  init_a=0  init_b=0  rst_a=off  rst_b=off  en_a=off  en_b=off  latency=1  write_mode_A=Read Before Write  write_mode_B=Read Before Write  dbl_ovrd=off  optimize=Speed  block_type=dpram
  wrlen : Outport
  epty : Outport  Port=2
  Ofullut3 : Outport  Port=3
  halffull : Outport  Port=4
  wires:
  Relational5/1 -> Ofullut3/1
  wrAddrCopy/1 -> L8_0_3/1
  Relational4/1 -> epty/1
  we/1 -> Gateway Out/1, wrAddrCopy/6
  rdaddress/1 -> L8_0_2/1
  Constant2/1 -> Relational4/2
  Relational1/1 -> halffull/1
  c_bool_3/1 -> wrAddrCopy/3
  c_uint10_2/1 -> wrAddrCopy/2
  L8_0_2/1 -> AddSub/2
  wrAddrCopy/2 -> Terminator2/1
  AddSub/1 -> wrlen/1, Relational1/1, Relational5/1, Relational4/1
  Constant3/1 -> Relational5/2
  Constant4/1 -> Relational1/2
  chan2/1 -> wrAddrCopy/4, Gateway Out2/1
  wraddr/1 -> Gateway Out1/1, wrAddrCopy/5
  L8_0_3/1 -> AddSub/1
  chan/1 -> wrAddrCopy/1
  Gateway Out2/1 -> Scope/3
  Gateway Out1/1 -> Scope/2
  Gateway Out/1 -> Scope/1

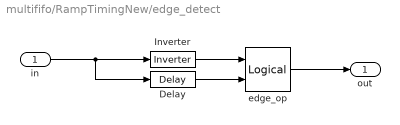
== system multififo/RampTimingNew/edge_detect ==
  in : Inport
  Delay : xbsIndex_r4/Delay  rst=off  infoeditControl=Selection of Reset will increase slice count due to use of real FFs and instead of SRLs  en=off  latency=1  dbl_ovrd=off  reg_retiming=off  block_type=delay
      settings: xl_area=[0, 0, 0, 0, 0, 0, 0]
  Inverter : xbsIndex_r4/Inverter  en=off  latency=0  dbl_ovrd=off  block_type=inv
      settings: xl_area=[0, 0, 0, 0, 0, 0, 0]
  edge_op : xbsIndex_r4/Logical  logical_function=NOR  inputs=2  en=off  latency=0  precision=Full  arith_type=Unsigned  n_bits=8  bin_pt=2  align_bp=on  dbl_ovrd=off  block_type=logical
      settings: xl_area=[0, 0, 0, 0, 0, 0, 0]
  out : Outport
  wires:
  Inverter/1 -> edge_op/1
  edge_op/1 -> out/1
  in/1 -> Inverter/1, Delay/1
  Delay/1 -> edge_op/2

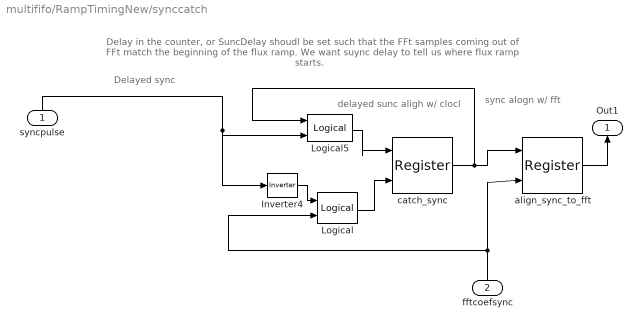
== system multififo/RampTimingNew/synccatch ==
  note: sync alogn w/ fft
  note: delayed
      | sunc
      | aligh w/ clocl
  note: Delay in the counter, or SuncDelay shoudl be set such that the
      | FFt samples coming out of FFt match the beginning of the flux ramp.
      | We want suync delay to tell us where flux ramp starts.
  note: Delayed sync
  syncpulse : Inport
  fftcoefsync : Inport  Port=2
  Inverter4 : xbsIndex_r4/Inverter  en=off  latency=0  dbl_ovrd=off  block_type=inv
  Logical : xbsIndex_r4/Logical  logical_function=AND  inputs=2  en=off  latency=0  precision=Full  arith_type=Unsigned  n_bits=16  bin_pt=0  align_bp=on  dbl_ovrd=off  block_type=logical
  Logical5 : xbsIndex_r4/Logical  logical_function=OR  inputs=2  en=off  latency=0  precision=Full  arith_type=Unsigned  n_bits=16  bin_pt=0  align_bp=on  dbl_ovrd=off  block_type=logical
  align_sync_to_fft : xbsIndex_r4/Register  init=0  rst=off  en=on  dbl_ovrd=off  block_type=register
  catch_sync : xbsIndex_r4/Register  init=0  rst=on  en=off  dbl_ovrd=off  block_type=register
  Out1 : Outport
  wires:
  syncpulse/1 -> Inverter4/1, Logical5/2
  fftcoefsync/1 -> Logical/2, align_sync_to_fft/2
  align_sync_to_fft/1 -> Out1/1
  Inverter4/1 -> Logical/1
  catch_sync/1 -> Logical5/1, align_sync_to_fft/1
  Logical5/1 -> catch_sync/1
  Logical/1 -> catch_sync/2
